simulink model "Assignment_1_V4_Final"  (R2022b)
settings: Solver=FixedStepAuto  StartTime=0.0  StopTime=10.0  FixedStep=1e-3  RelTol=1e-3  EnableMultiTasking=on
undefined symbols (not defined in the file): D0, D1, D10, D11, D12, D13, D2, D3, D4, D5, D6, D7, D8, D9, PTA0, PTA1, PTA2, PTB23, PTB9, PTC16, PTC17, PTC2, PTC3, PTC4, PTD0, PTD1, PTD2, PTD3
libraries: frdmk64flib x14
settings Model: ExtModeTrigDuration=5  Creator=annan  LastModifiedBy=tjism
settings OptimizationCC: EnhancedBackFolding=on  PassReuseOutputArgsAs=Individual arguments  ZeroExternalMemoryAtStartup=off  ZeroInternalMemoryAtStartup=off  MaxStackSize=64  OptimizeBlockOrder=speed  DifferentSizesBufferReuse=on  OptimizationCustomize=off  EfficientTunableParamExpr=on
settings DebuggingCC: ParameterTunabilityLossMsg=error
settings HardwareCC: ProdBitPerPointer=32  ProdBitPerSizeT=32  ProdBitPerPtrDiffT=32  ProdLargestAtomicInteger=Long  ProdLargestAtomicFloat=Double  ProdWordSize=32  ProdHWDeviceType=ARM Compatible->ARM Cortex
settings SFSimCC: MATLABDynamicMemAlloc=off
settings RTWCC: Description=Embedded Coder  SystemTargetFile=ert.tlc  HardwareBoard=NXP FRDM-K64F  TLCOptions="-aInlineSetEventsForThisBaseRateFcn=TLC_FALSE -aSuppressMultiTaskScheduler=TLC_FALSE  -aRateBasedStepFcn=0"  TemplateMakefile=ert_default_tmf  Toolchain=GNU Tools for ARM Embedded Processors
settings CodeAppCC: ForceParamTrailComments=on  IgnoreCustomStorageClasses=off  OperatorAnnotations=on  SimulinkDataObjDesc=on  SFDataObjDesc=on  InsertBlockDesc=on
settings ERTTargetCC: ExtModeTransport=4  ExtModeMexFile=sendToCommService

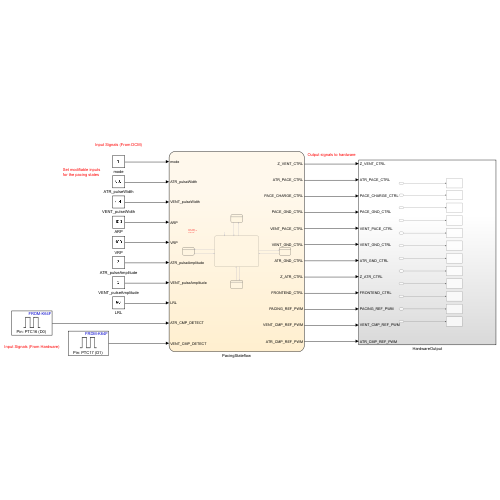
[thumbnail: Simulink's stored preview of the top-level diagram]
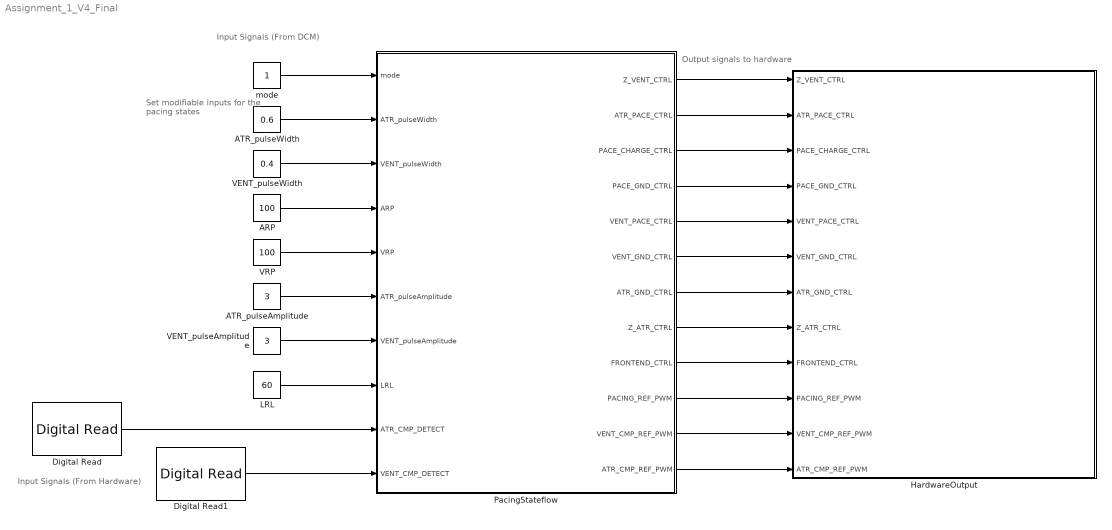
== system Assignment_1_V4_Final ==
  note: Set modifiable inputs for the pacing states
  note: Input Signals (From Hardware)
  note: Input Signals (From DCM)
  note: Output signals to hardware
  ARP : Constant  Value=100
  ATR_pulseAmplitude : Constant  Value=3
  ATR_pulseWidth : Constant  Value=0.6  OutDataTypeStr=double
  Digital Read : frdmk64flib/Digital Read  Whichpin=PTC16 (D0)  SampleTime=-1
  Digital Read1 : frdmk64flib/Digital Read  Whichpin=PTC17 (D1)  SampleTime=-1
  HardwareOutput : Subsystem
  LRL : Constant  Value=60
  PacingStateflow : Stateflow chart  TreatAsAtomicUnit=on
      settings: PortSchema="{\"entries\":[{\"content\":{\"sides\":[{\"content\":{\"connectorIds\":[\"In1\",\"In2\",\"In3\",\"In5\",\"In4\",\"In8\",\"In7\",\"In6\",\"In9\",\"In10\"]},\"type\":\"ConnectorPlacement.EquallySpacedRectSide\",\"uuid\":\"576c6451-25f7-4bf9-8ba9-b62bfe0038eb\"},{\"content\":{\"connectorIds\":[\"Out1\",\"Out2\",\"Out3\",\"Out4\",\"Out5\",\"Out6\",\"Out7\",\"Out8\",\"Out9\",\"Out10\",\"Out11\",\"Out12\"],\"side\":\"RIGHT\"},\"type\":\"ConnectorPlacement.EquallySpacedRectSide\",\"uuid\":\"13f5cd1e-83b9-45c9-ae47-e36f7742cdf1\"},{\"content\":{\"connectorIds\":[],\"side\":\"TOP\"},\"type\":\"ConnectorPlacement.EquallySpacedRectSide\",\"uuid\":\"e0eaa1cf-7eb4-4233-8973-4ce0d50eac65\"}]},\"type\":\"ConnectorPlacement.EquallySpacedConnector\",\"uuid\":\"6190d1e8-de04-4ebf-bfa3-72cd0ed3652a\"}],\"packageUris\":[\"http://schema.mathworks.com/mf0/Connector/R2020b\"],\"version\":\"1.0\"}"
  VENT_pulseAmplitude : Constant  Value=3
  VENT_pulseWidth : Constant  Value=0.4
  VRP : Constant  Value=100  OutDataTypeStr=double
  mode : Constant  OutDataTypeStr=int32
  wires:
  PacingStateflow/1(Z_VENT_CTRL) -> HardwareOutput/1(Z_VENT_CTRL)
  PacingStateflow/2(ATR_PACE_CTRL) -> HardwareOutput/2(ATR_PACE_CTRL)
  PacingStateflow/3(PACE_CHARGE_CTRL) -> HardwareOutput/3(PACE_CHARGE_CTRL)
  PacingStateflow/4(PACE_GND_CTRL) -> HardwareOutput/4(PACE_GND_CTRL)
  PacingStateflow/5(VENT_PACE_CTRL) -> HardwareOutput/5(VENT_PACE_CTRL)
  PacingStateflow/6(VENT_GND_CTRL) -> HardwareOutput/6(VENT_GND_CTRL)
  PacingStateflow/7(ATR_GND_CTRL) -> HardwareOutput/7(ATR_GND_CTRL)
  PacingStateflow/8(Z_ATR_CTRL) -> HardwareOutput/8(Z_ATR_CTRL)
  LRL/1 -> PacingStateflow/6(LRL)
  VRP/1 -> PacingStateflow/4(VRP)
  ATR_pulseWidth/1 -> PacingStateflow/2(ATR_pulseWidth)
  mode/1 -> PacingStateflow/1(mode)
  Digital Read/1 -> PacingStateflow/9(ATR_CMP_DETECT)
  Digital Read1/1 -> PacingStateflow/10(VENT_CMP_DETECT)
  PacingStateflow/10(PACING_REF_PWM) -> HardwareOutput/10(PACING_REF_PWM)
  VENT_pulseAmplitude/1 -> PacingStateflow/7(VENT_pulseAmplitude)
  PacingStateflow/9(FRONTEND_CTRL) -> HardwareOutput/9(FRONTEND_CTRL)
  PacingStateflow/11(VENT_CMP_REF_PWM) -> HardwareOutput/11(VENT_CMP_REF_PWM)
  PacingStateflow/12(ATR_CMP_REF_PWM) -> HardwareOutput/12(ATR_CMP_REF_PWM)
  VENT_pulseWidth/1 -> PacingStateflow/3(VENT_pulseWidth)
  ARP/1 -> PacingStateflow/5(ARP)
  ATR_pulseAmplitude/1 -> PacingStateflow/8(ATR_pulseAmplitude)

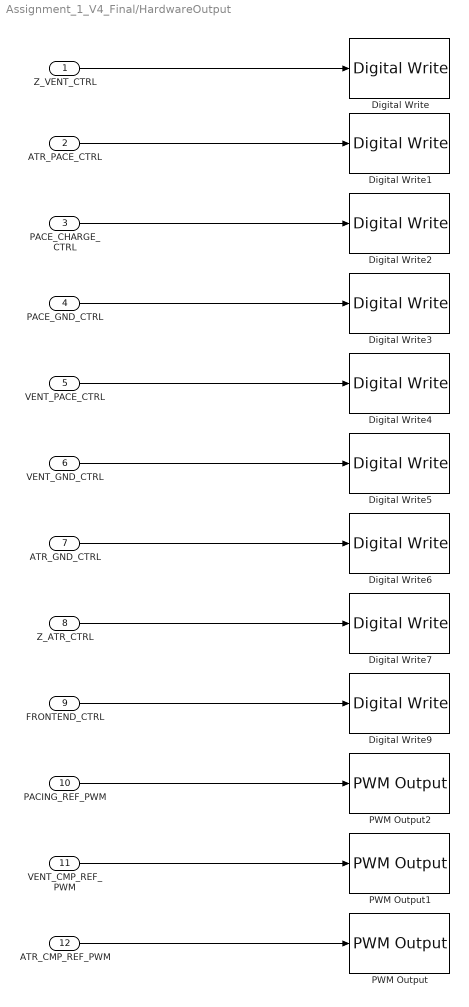
== system Assignment_1_V4_Final/HardwareOutput ==
  Z_VENT_CTRL : Inport
  ATR_PACE_CTRL : Inport  Port=2
  PACE_CHARGE_CTRL : Inport  Port=3
  PACE_GND_CTRL : Inport  Port=4
  VENT_PACE_CTRL : Inport  Port=5
  VENT_GND_CTRL : Inport  Port=6
  ATR_GND_CTRL : Inport  Port=7
  Z_ATR_CTRL : Inport  Port=8
  FRONTEND_CTRL : Inport  Port=9
  PACING_REF_PWM : Inport  Port=10
  VENT_CMP_REF_PWM : Inport  Port=11
  ATR_CMP_REF_PWM : Inport  Port=12
  Digital Write : frdmk64flib/Digital Write  Whichpin=PTC3 (D7)
  Digital Write1 : frdmk64flib/Digital Write  Whichpin=PTA0 (D8)
  Digital Write2 : frdmk64flib/Digital Write  Whichpin=PTB9 (D2)
  Digital Write3 : frdmk64flib/Digital Write  Whichpin=PTD0 (D10)
  Digital Write4 : frdmk64flib/Digital Write  Whichpin=PTC4 (D9)
  Digital Write5 : frdmk64flib/Digital Write  Whichpin=PTD3 (D12)
  Digital Write6 : frdmk64flib/Digital Write  Whichpin=PTD2 (D11)
  Digital Write7 : frdmk64flib/Digital Write  Whichpin=PTB23 (D4)
  Digital Write9 : frdmk64flib/Digital Write  Whichpin=PTD1 (D13)
  PWM Output : frdmk64flib/PWM Output  Whichpin=PTC2 (D6)  InitialFrequency=2000  InitialDutyCycle=0
  PWM Output1 : frdmk64flib/PWM Output  Whichpin=PTA1 (D3)  InitialFrequency=2000  InitialDutyCycle=0
  PWM Output2 : frdmk64flib/PWM Output  Whichpin=PTA2 (D5)  InitialFrequency=2000  InitialDutyCycle=0
  wires:
  Z_VENT_CTRL/1 -> Digital Write/1
  ATR_PACE_CTRL/1 -> Digital Write1/1
  PACE_CHARGE_CTRL/1 -> Digital Write2/1
  PACE_GND_CTRL/1 -> Digital Write3/1
  VENT_PACE_CTRL/1 -> Digital Write4/1
  VENT_GND_CTRL/1 -> Digital Write5/1
  ATR_GND_CTRL/1 -> Digital Write6/1
  Z_ATR_CTRL/1 -> Digital Write7/1
  PACING_REF_PWM/1 -> PWM Output2/1
  FRONTEND_CTRL/1 -> Digital Write9/1
  VENT_CMP_REF_PWM/1 -> PWM Output1/1
  ATR_CMP_REF_PWM/1 -> PWM Output/1

== stateflow chart Assignment_1_V4_Final/PacingStateflow ==
  state AOO
    note: This transition ensures we reulate the time spent in each state and pulse at the proper rate. This is the time it takes per one pulse, as determined by the LRL, minus the time spent pulsing.
    note: Atrial mode with no sensing.
        | Constant BPM output.
    state AOO_Charge
      entry:
      PACING_REF_PWM = 100*(ATR_pulseAmplitude/double(5.0));
      % Charging C22
      ATR_PACE_CTRL = false;
      VENT_PACE_CTRL = false;
      PACE_CHARGE_CTRL = true;
      PACE_GND_CTRL = true;
      Z_ATR_CTRL = false;
      Z_VENT_CTRL = false;
      % Discharging C21
      ATR_GND_CTRL = true;
      VENT_GND_CTRL = false;
    state AOO_Discharge
      entry:
      PACE_CHARGE_CTRL = false;
      PACE_GND_CTRL = true;
      ATR_PACE_CTRL = true;
      ATR_GND_CTRL = false;
      Z_ATR_CTRL = false;
      Z_VENT_CTRL = false;
      VENT_GND_CTRL = false;
      VENT_PACE_CTRL = false;
    note: After discharging C22 into the atrium for the
        | desired pulse width, return to the default state
        | to charge C22 and discharge C21.
    AOO_Charge -> AOO_Discharge : [after(pulseTime - ATR_pulseWidth, msec)]
    (default) -> AOO_Charge
    AOO_Discharge -> AOO_Charge : [after(ATR_pulseWidth,msec)]
  note: enter state depending on mode set
  state Entry_State
    entry:
    VENT_PACE_CTRL = false;
    ATR_PACE_CTRL = false;
    VENT_GND_CTRL = false;
    ATR_GND_CTRL = false;
    PACE_GND_CTRL = false;
    PACE_CHARGE_CTRL = false;
    FRONTEND_CTRL = false;
    VENT_CMP_REF_PWM = 0;
    ATR_CMP_REF_PWM = 0;
    Z_ATR_CTRL = false;
    Z_VENT_CTRL = false;
    pulseTime = 60000/LRL;
  state AAI
    note: This state is responsible for charging the pacing circuitry and preparing the system for either sensing or pacing
    note: Moves to the sensing state after the atrial refractory period to monitor atrial activity
    state AAI_Sensing
      entry:
      % Charging C22
      FRONTEND_CTRL = true;
      ATR_CMP_REF_PWM = 55;
      PACING_REF_PWM = 100*(ATR_pulseAmplitude / 5.0);
      VENT_PACE_CTRL = false;
      ATR_PACE_CTRL = false;
      PACE_CHARGE_CTRL = true;
      % Discharging C21
      PACE_GND_CTRL = true;
      ATR_GND_CTRL = true;
      VENT_GND_CTRL = false;
    state AAI_Charge
      entry:
      % Charging C22
      FRONTEND_CTRL = true;
      ATR_CMP_REF_PWM = 55;
      PACING_REF_PWM = 100*(ATR_pulseAmplitude / 5.0);
      VENT_PACE_CTRL = false;
      ATR_PACE_CTRL = false;
      PACE_CHARGE_CTRL = true;
      % Discharging C21
      PACE_GND_CTRL = true;
      ATR_GND_CTRL = true;
      VENT_GND_CTRL = false;
    note: Returns to the charging state if atrial activity is detected
    state AAI_Discharge
      entry:
      PACE_CHARGE_CTRL = false;
      PACE_GND_CTRL = true;
      VENT_PACE_CTRL = false;
      ATR_PACE_CTRL = true;
      ATR_GND_CTRL = false;
      VENT_GND_CTRL = false;
    note: Moves to the discharge state to deliver a pacing pulse after the specified time if no natural atrial signal is detected
    note: after the above calculated wait time, go into the recharge state
    (default) -> AAI_Charge
    AAI_Charge -> AAI_Sensing : after(ARP, msec)
    AAI_Sensing -> AAI_Charge [order 1] : [ATR_CMP_DETECT == true]
    AAI_Discharge -> AAI_Charge : after(ATR_pulseWidth, msec)
    AAI_Sensing -> AAI_Discharge [order 2] : after(pulseTime - ARP - ATR_pulseWidth, msec)
  state VOO
    note: This transition ensures we reulate the time spent in each state and pulse at the proper rate. This is the time it takes per one pulse, as determined by the LRL, minus the time spent pulsing.
    note: Ventricle mode with no sensing.
        | Constant BPM output.
    state VOO_Charge
      entry:
      PACING_REF_PWM = 100*(ATR_pulseAmplitude/double(5.0));
      % Charging C22
      ATR_PACE_CTRL = false;
      VENT_PACE_CTRL = false;
      PACE_CHARGE_CTRL = true;
      PACE_GND_CTRL = true;
      Z_ATR_CTRL = false;
      Z_VENT_CTRL = false;
      % Discharging C21
      ATR_GND_CTRL = false;
      VENT_GND_CTRL = true;
    state VOO_Discharge
      entry:
      PACE_CHARGE_CTRL = false;
      PACE_GND_CTRL = true;
      ATR_PACE_CTRL = false;
      ATR_GND_CTRL = false;
      Z_ATR_CTRL = false;
      Z_VENT_CTRL = false;
      VENT_GND_CTRL = false;
      VENT_PACE_CTRL = true;
    note: After discharging C22 into the ventricle for the
        | desired pulse width, return to the default state
        | to charge C22 and discharge C21.
    VOO_Charge -> VOO_Discharge : [after(pulseTime - VENT_pulseWidth, msec)]
    (default) -> VOO_Charge
    VOO_Discharge -> VOO_Charge : [after(VENT_pulseWidth,msec)]
  state VVI
    note: This state is responsible for charging the pacing circuitry and preparing the system for either sensing or pacing
    note: Moves to the sensing state after the ventricular refractory period to monitor ventricle activity
    state VVI_Charge
      entry:
      % Charging C22
      FRONTEND_CTRL = true;
      VENT_CMP_REF_PWM = 53;
      PACING_REF_PWM = 100*(VENT_pulseAmplitude / 5.0);
      VENT_PACE_CTRL = false;
      ATR_PACE_CTRL = false;
      PACE_CHARGE_CTRL = true;
      % Discharging C21
      PACE_GND_CTRL = true;
      ATR_GND_CTRL = false;
      VENT_GND_CTRL = true;
    state VVI_Sensing
      entry:
      % Charging C22
      FRONTEND_CTRL = true;
      VENT_CMP_REF_PWM = 53;
      PACING_REF_PWM = 100*(VENT_pulseAmplitude / 5.0);
      VENT_PACE_CTRL = false;
      ATR_PACE_CTRL = false;
      PACE_CHARGE_CTRL = true;
      % Discharging C21
      PACE_GND_CTRL = true;
      ATR_GND_CTRL = false;
      VENT_GND_CTRL = true;
    note: Returns to the charging state if ventricle activity is detected
    state VVI_Discharge
      entry:
      PACE_CHARGE_CTRL = false;
      PACE_GND_CTRL = true;
      VENT_PACE_CTRL = true;
      ATR_PACE_CTRL = false;
      ATR_GND_CTRL = false;
      VENT_GND_CTRL = false;
    note: Moves to the discharge state to deliver a pacing pulse after the specified time if no natural ventricular signal is detected
    (default) -> VVI_Charge
    VVI_Charge -> VVI_Sensing : after(VRP, msec)
    VVI_Sensing -> VVI_Charge [order 1] : [VENT_CMP_DETECT == true]
    VVI_Discharge -> VVI_Charge : after(VENT_pulseWidth, msec)
    VVI_Sensing -> VVI_Discharge [order 2] : after(pulseTime - VRP - VENT_pulseWidth, msec)
  AOO -> Entry_State : [mode ~= 1]
  Entry_State -> AOO [order 1] : [mode == 1]
  (default) -> Entry_State
  Entry_State -> AAI [order 4] : [mode == 3]
  Entry_State -> VOO [order 2] : [mode == 2]
  AAI -> Entry_State : [mode ~= 3]
  VOO -> Entry_State : [mode ~= 2]
  VVI -> Entry_State : [mode ~= 4]
  Entry_State -> VVI [order 3] : [mode == 4]
  data: mode input int32; ATR_pulseWidth input double; VENT_pulseWidth input; VRP input double; ARP input; LRL input double; VENT_pulseAmplitude input; ATR_pulseAmplitude input; ATR_CMP_DETECT input; VENT_CMP_DETECT input boolean; Z_VENT_CTRL output boolean; ATR_PACE_CTRL output boolean; PACE_CHARGE_CTRL output boolean; PACE_GND_CTRL output boolean; VENT_PACE_CTRL output boolean; VENT_GND_CTRL output boolean; ATR_GND_CTRL output boolean; Z_ATR_CTRL output boolean; FRONTEND_CTRL output; PACING_REF_PWM output; VENT_CMP_REF_PWM output; ATR_CMP_REF_PWM output; pulseTime local
